simulink library "REORDER"  (R2019a)
settings: Solver=VariableStepAuto  StartTime=0.0  StopTime=10.0  RelTol=1e-3
libraries: xbsIndex_r4 x2
settings Model: Creator=Ross Donnachie  LastModifiedBy=Ross Donnachie

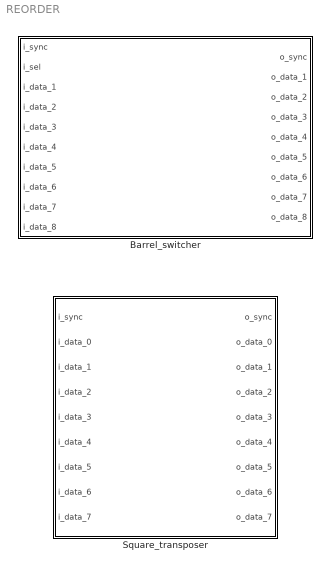
== system REORDER ==
  Barrel_switcher : Subsystem  mask{number_of_ports_2exp=3, port_bit_width=4, async=on}
      mask prompts: number_of_ports_2exp "Number of inputs (2^?):"; port_bit_width "Port bit-width:"; async "Asynchronous operation"
      mask init:
      | Simulink.Block.eval([gcb, '/barrel_switcher']);
      | 
      | knit_subsystem_to_blackbox('barrel_switcher');
  Square_transposer : Subsystem  mask{number_of_ports_2exp=3, port_bit_width=4, async=off}
      mask prompts: number_of_ports_2exp "Number of inputs (2^?):"; port_bit_width "Port bit-width:"; async "Asynchronous operation"
      mask init:
      | Simulink.Block.eval([gcb, '/square_transposer']);
      | 
      | knit_subsystem_to_blackbox('square_transposer');

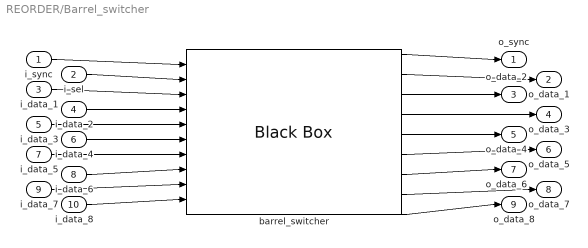
== system REORDER/Barrel_switcher ==
  i_sync : Inport
  i_sel : Inport  Port=2
  i_data_1 : Inport  Port=3
  i_data_2 : Inport  Port=4
  i_data_3 : Inport  Port=5
  i_data_4 : Inport  Port=6
  i_data_5 : Inport  Port=7
  i_data_6 : Inport  Port=8
  i_data_7 : Inport  Port=9
  i_data_8 : Inport  Port=10
  barrel_switcher : xbsIndex_r4/Black Box  init_code=barrel_switcher_config  sim_method=ISE Simulator  verbose=on  block_type=blackbox2
  o_sync : Outport
  o_data_1 : Outport  Port=2
  o_data_2 : Outport  Port=3
  o_data_3 : Outport  Port=4
  o_data_4 : Outport  Port=5
  o_data_5 : Outport  Port=6
  o_data_6 : Outport  Port=7
  o_data_7 : Outport  Port=8
  o_data_8 : Outport  Port=9
  wires:
  i_sync/1 -> barrel_switcher/1
  i_sel/1 -> barrel_switcher/2
  i_data_1/1 -> barrel_switcher/3
  i_data_2/1 -> barrel_switcher/4
  i_data_3/1 -> barrel_switcher/5
  i_data_4/1 -> barrel_switcher/6
  i_data_5/1 -> barrel_switcher/7
  i_data_6/1 -> barrel_switcher/8
  i_data_7/1 -> barrel_switcher/9
  i_data_8/1 -> barrel_switcher/10
  barrel_switcher/1 -> o_sync/1
  barrel_switcher/2 -> o_data_1/1
  barrel_switcher/3 -> o_data_2/1
  barrel_switcher/4 -> o_data_3/1
  barrel_switcher/5 -> o_data_4/1
  barrel_switcher/6 -> o_data_5/1
  barrel_switcher/7 -> o_data_6/1
  barrel_switcher/8 -> o_data_7/1
  barrel_switcher/9 -> o_data_8/1

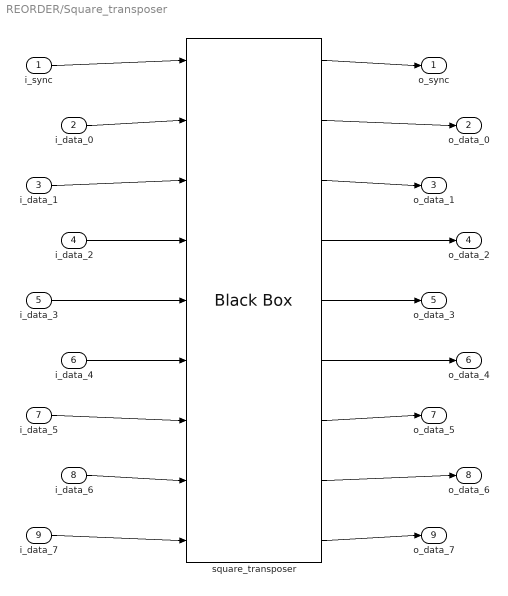
== system REORDER/Square_transposer ==
  i_sync : Inport
  i_data_0 : Inport  Port=2
  i_data_1 : Inport  Port=3
  i_data_2 : Inport  Port=4
  i_data_3 : Inport  Port=5
  i_data_4 : Inport  Port=6
  i_data_5 : Inport  Port=7
  i_data_6 : Inport  Port=8
  i_data_7 : Inport  Port=9
  square_transposer : xbsIndex_r4/Black Box  init_code=square_transposer_config  sim_method=ISE Simulator  verbose=on  block_type=blackbox2
  o_sync : Outport
  o_data_0 : Outport  Port=2
  o_data_1 : Outport  Port=3
  o_data_2 : Outport  Port=4
  o_data_3 : Outport  Port=5
  o_data_4 : Outport  Port=6
  o_data_5 : Outport  Port=7
  o_data_6 : Outport  Port=8
  o_data_7 : Outport  Port=9
  wires:
  i_sync/1 -> square_transposer/1
  i_data_0/1 -> square_transposer/2
  i_data_1/1 -> square_transposer/3
  i_data_2/1 -> square_transposer/4
  i_data_3/1 -> square_transposer/5
  i_data_4/1 -> square_transposer/6
  i_data_5/1 -> square_transposer/7
  i_data_6/1 -> square_transposer/8
  i_data_7/1 -> square_transposer/9
  square_transposer/1 -> o_sync/1
  square_transposer/2 -> o_data_0/1
  square_transposer/3 -> o_data_1/1
  square_transposer/4 -> o_data_2/1
  square_transposer/5 -> o_data_3/1
  square_transposer/6 -> o_data_4/1
  square_transposer/7 -> o_data_5/1
  square_transposer/8 -> o_data_6/1
  square_transposer/9 -> o_data_7/1
